simulink model "signal_operations_simulink"  (R2024b)
settings: Solver=VariableStepAuto  StartTime=0.0  StopTime=10.0  RelTol=1e-3
settings Model: Creator=LENOVO  LastModifiedBy=LENOVO

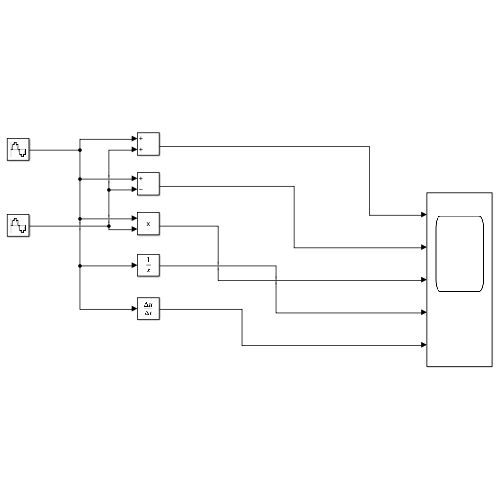
[thumbnail: Simulink's stored preview of the top-level diagram]
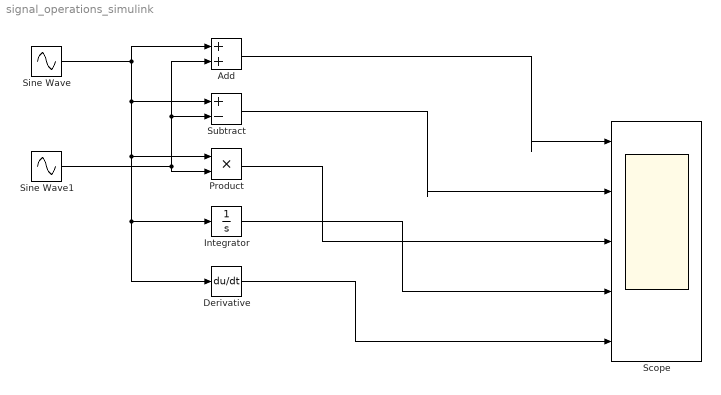
== system signal_operations_simulink ==
  Add : Sum
  Derivative : Derivative
  Integrator : Integrator
  Product : Product
  Scope : Scope  NumInputPorts=5
  Sine Wave : Sin  SampleTime=0.001
  Sine Wave1 : Sin  Amplitude=3  SampleTime=0.001
  Subtract : Sum  Inputs=+-
  wires:
  Sine Wave/1 -> Derivative/1, Integrator/1, Product/1, Subtract/1, Add/1
  Sine Wave1/1 -> Subtract/2, Add/2, Product/2
  Add/1 -> Scope/1
  Integrator/1 -> Scope/4
  Derivative/1 -> Scope/5
  Product/1 -> Scope/3
  Subtract/1 -> Scope/2
